simulink model "sl_quadcopter_tres_poster"  (R2014a)
settings: Solver=ode45  StartTime=0.0  StopTime=20  MaxStep=0.1  RelTol=1e-3
InitFcn:
  | % load parameters of the default quadrotor
  | disp('Quadrotor parameters loaded by InitFcn')
  | mdl_quadcopter
undefined symbols (not defined in the file or in its folder): quad
libraries: tres_simulink_blockset x5, roblocks x2
settings Model: Creator=corkep  LastModifiedBy=matteo
settings DataIOCC: SignalLoggingSaveFormat=ModelDataLogs
settings OptimizationCC: ExpressionDepthLimit=2147483647
settings DebuggingCC: UnderspecifiedInitializationDetection=Classic  FcnCallInpInsideContextMsg=EnableAllAsWarning  StateNameClashWarn=warning
settings GRTTargetCC: CombineOutputUpdateFcns=off  GRTInterface=on

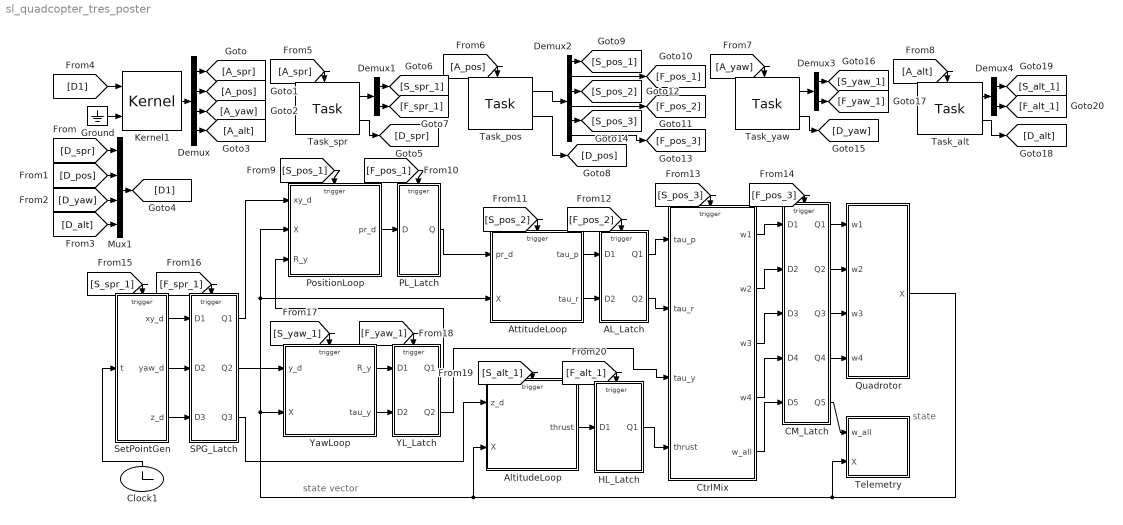
== system sl_quadcopter_tres_poster ==
  note: state
  note: state vector
  AL_Latch : Subsystem  TreatAsAtomicUnit=on
  AltitudeLoop : Subsystem
  AttitudeLoop : Subsystem
  CM_Latch : Subsystem  TreatAsAtomicUnit=on
  Clock1 : Clock
  CtrlMix : Subsystem
  Demux : Demux
  Demux1 : Demux  Outputs=2
  Demux2 : Demux  Outputs=6
  Demux3 : Demux  Outputs=2
  Demux4 : Demux  Outputs=2
  Ground : Ground
  HL_Latch : Subsystem  TreatAsAtomicUnit=on
  Kernel1 : tres_simulink_blockset/Kernel  taskset_descr_name=task_set_descr  scheduling_policy=FIXED_PRIORITY  dead_miss_rule=Continue  time_res=Milli_Seconds  core_num=1  under_engine=RTSIM
  Mux1 : Mux
  PL_Latch : Subsystem  TreatAsAtomicUnit=on
  PositionLoop : Subsystem
  Quadrotor : Subsystem
  SPG_Latch : Subsystem  TreatAsAtomicUnit=on
  SetPointGen : Subsystem
  Task_alt : tres_simulink_blockset/Task  conf_name=alt_instrs
  Task_pos : tres_simulink_blockset/Task  conf_name=att_instrs
  Task_spr : tres_simulink_blockset/Task  conf_name=spr_instrs
  Task_yaw : tres_simulink_blockset/Task  conf_name=yaw_instrs
  Telemetry : Subsystem
  YL_Latch : Subsystem  TreatAsAtomicUnit=on
  YawLoop : Subsystem
  wires:
  SetPointGen/1(xy_d) -> SPG_Latch/1(D1)
  Clock1/1 -> SetPointGen/1(t)
  SetPointGen/2(yaw_d) -> SPG_Latch/2(D2)
  SetPointGen/3(z_d) -> SPG_Latch/3(D3)
  SPG_Latch/1(Q1) -> PositionLoop/1(xy_d)
  SPG_Latch/2(Q2) -> YawLoop/1(y_d)
  SPG_Latch/3(Q3) -> AltitudeLoop/1(z_d)
  YawLoop/1(R_y) -> YL_Latch/1(D1)
  YL_Latch/1(Q1) -> PositionLoop/3(R_y)
  YawLoop/2(tau_y) -> YL_Latch/2(D2)
  YL_Latch/2(Q2) -> CtrlMix/3(tau_y)
  AltitudeLoop/1(thrust) -> HL_Latch/1(D1)
  HL_Latch/1(Q1) -> CtrlMix/4(thrust)
  PositionLoop/1(pr_d) -> PL_Latch/1(D)
  PL_Latch/1(Q) -> AttitudeLoop/1(pr_d)
  AttitudeLoop/1(tau_p) -> AL_Latch/1(D1)
  AttitudeLoop/2(tau_r) -> AL_Latch/2(D2)
  AL_Latch/1(Q1) -> CtrlMix/1(tau_p)
  AL_Latch/2(Q2) -> CtrlMix/2(tau_r)
  CtrlMix/1(w1) -> CM_Latch/1(D1)
  CtrlMix/2(w2) -> CM_Latch/2(D2)
  CtrlMix/3(w3) -> CM_Latch/3(D3)
  CtrlMix/4(w4) -> CM_Latch/4(D4)
  CtrlMix/5(w_all) -> CM_Latch/5(D5)
  CM_Latch/5(Q5) -> Telemetry/1(w_all)
  Ground/1 -> Kernel1/2
  [D_spr] -> Mux1/1
  [D_pos] -> Mux1/2
  [D_yaw] -> Mux1/3
  [D_alt] -> Mux1/4
  Kernel1/1 -> Demux/1
  Demux/1 -> [A_spr]
  Demux/2 -> [A_pos]
  Demux/3 -> [A_yaw]
  Demux/4 -> [A_alt]
  Mux1/1 -> [D1]
  [D1] -> Kernel1/1
  [A_spr] -> Task_spr/Trigger
  Task_spr/1 -> Demux1/1
  Task_spr/2 -> [D_spr]
  Demux1/1 -> [S_spr_1]
  Demux1/2 -> [F_spr_1]
  [A_pos] -> Task_pos/Trigger
  Task_pos/1 -> Demux2/1
  Task_pos/2 -> [D_pos]
  Demux2/1 -> [S_pos_1]
  Demux2/2 -> [F_pos_1]
  Demux2/3 -> [S_pos_2]
  Demux2/4 -> [F_pos_2]
  Demux2/5 -> [S_pos_3]
  Demux2/6 -> [F_pos_3]
  [A_yaw] -> Task_yaw/Trigger
  Task_yaw/1 -> Demux3/1
  Task_yaw/2 -> [D_yaw]
  Demux3/1 -> [S_yaw_1]
  Demux3/2 -> [F_yaw_1]
  [A_alt] -> Task_alt/Trigger
  Task_alt/1 -> Demux4/1
  Task_alt/2 -> [D_alt]
  Demux4/1 -> [S_alt_1]
  Demux4/2 -> [F_alt_1]
  [S_pos_1] -> PositionLoop/Trigger
  [F_pos_1] -> PL_Latch/Trigger
  [F_pos_2] -> AL_Latch/Trigger
  [S_pos_2] -> AttitudeLoop/Trigger
  [S_yaw_1] -> YawLoop/Trigger
  [F_yaw_1] -> YL_Latch/Trigger
  [S_spr_1] -> SetPointGen/Trigger
  [F_spr_1] -> SPG_Latch/Trigger
  [S_pos_3] -> CtrlMix/Trigger
  [F_pos_3] -> CM_Latch/Trigger
  [S_alt_1] -> AltitudeLoop/Trigger
  [F_alt_1] -> HL_Latch/Trigger
  Quadrotor/1(X) -> Telemetry/2(X), YawLoop/2(X), AttitudeLoop/2(X), PositionLoop/2(X), AltitudeLoop/2(X)
  CM_Latch/1(Q1) -> Quadrotor/1(w1)
  CM_Latch/2(Q2) -> Quadrotor/2(w2)
  CM_Latch/3(Q3) -> Quadrotor/3(w3)
  CM_Latch/4(Q4) -> Quadrotor/4(w4)

== system sl_quadcopter_tres_poster/AL_Latch ==
  D1 : Inport
  D2 : Inport  Port=2
  function : TriggerPort  TriggerType=function-call
  Q1 : Outport
  Q2 : Outport  Port=2
  wires:
  D1/1 -> Q1/1
  D2/1 -> Q2/1

== system sl_quadcopter_tres_poster/AltitudeLoop ==
  z_d : Inport
  X : Inport  Port=2
  function : TriggerPort  TriggerType=function-call  PortDimensions=1
  Subsystem : Subsystem
  thrust : Outport
  wires:
  X/1 -> Subsystem/2(In2)
  z_d/1 -> Subsystem/1(In1)
  Subsystem/1(Out1) -> thrust/1

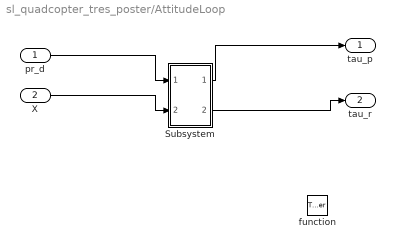
== system sl_quadcopter_tres_poster/AttitudeLoop ==
  pr_d : Inport
  X : Inport  Port=2
  function : TriggerPort  TriggerType=function-call  PortDimensions=1
  Subsystem : Subsystem
  tau_p : Outport
  tau_r : Outport  Port=2
  wires:
  Subsystem/1(Out1) -> tau_p/1
  pr_d/1 -> Subsystem/1(In1)
  Subsystem/2(Out2) -> tau_r/1
  X/1 -> Subsystem/2(In2)

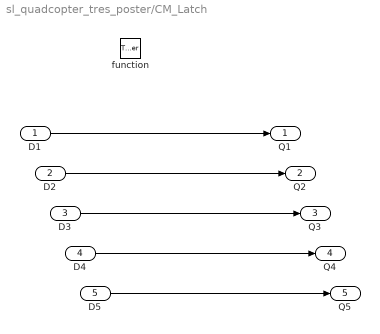
== system sl_quadcopter_tres_poster/CM_Latch ==
  D1 : Inport
  D2 : Inport  Port=2
  D3 : Inport  Port=3
  D4 : Inport  Port=4
  D5 : Inport  Port=5
  function : TriggerPort  TriggerType=function-call
  Q1 : Outport
  Q2 : Outport  Port=2
  Q3 : Outport  Port=3
  Q4 : Outport  Port=4
  Q5 : Outport  Port=5
  wires:
  D1/1 -> Q1/1
  D2/1 -> Q2/1
  D3/1 -> Q3/1
  D4/1 -> Q4/1
  D5/1 -> Q5/1

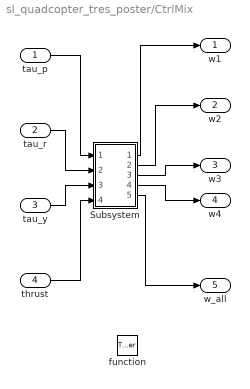
== system sl_quadcopter_tres_poster/CtrlMix ==
  tau_p : Inport
  tau_r : Inport  Port=2
  tau_y : Inport  Port=3
  thrust : Inport  Port=4
  function : TriggerPort  TriggerType=function-call  PortDimensions=1
  Subsystem : Subsystem
  w1 : Outport
  w2 : Outport  Port=2
  w3 : Outport  Port=3
  w4 : Outport  Port=4
  w_all : Outport  Port=5
  wires:
  Subsystem/1(Out1) -> w1/1
  tau_p/1 -> Subsystem/1(In1)
  Subsystem/2(Out2) -> w2/1
  tau_r/1 -> Subsystem/2(In2)
  Subsystem/3(Out3) -> w3/1
  tau_y/1 -> Subsystem/3(In3)
  Subsystem/4(Out4) -> w4/1
  thrust/1 -> Subsystem/4(In4)
  Subsystem/5(Out5) -> w_all/1

== system sl_quadcopter_tres_poster/HL_Latch ==
  D1 : Inport
  function : TriggerPort  TriggerType=function-call
  Q1 : Outport
  wires:
  D1/1 -> Q1/1

== system sl_quadcopter_tres_poster/PL_Latch ==
  D : Inport
  function : TriggerPort  TriggerType=function-call
  Q : Outport
  wires:
  D/1 -> Q/1

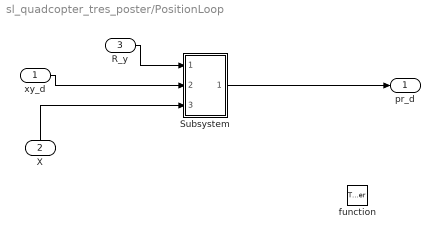
== system sl_quadcopter_tres_poster/PositionLoop ==
  xy_d : Inport
  X : Inport  Port=2
  R_y : Inport  Port=3
  function : TriggerPort  TriggerType=function-call  PortDimensions=1
  Subsystem : Subsystem
  pr_d : Outport
  wires:
  xy_d/1 -> Subsystem/2(In2)
  Subsystem/1(Out1) -> pr_d/1
  R_y/1 -> Subsystem/1(R_y)
  X/1 -> Subsystem/3(In3)

== system sl_quadcopter_tres_poster/Quadrotor ==
  w1 : Inport
  w2 : Inport  Port=2
  w3 : Inport  Port=3
  w4 : Inport  Port=4
  Quadrotor : roblocks/Dynamics/Quadrotor  quad=quad
  X : Outport
  wires:
  w1/1 -> Quadrotor/1
  w2/1 -> Quadrotor/2
  w3/1 -> Quadrotor/3
  w4/1 -> Quadrotor/4
  Quadrotor/1 -> X/1

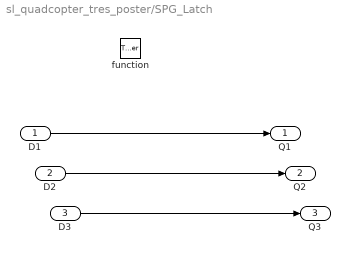
== system sl_quadcopter_tres_poster/SPG_Latch ==
  D1 : Inport
  D2 : Inport  Port=2
  D3 : Inport  Port=3
  function : TriggerPort  TriggerType=function-call
  Q1 : Outport
  Q2 : Outport  Port=2
  Q3 : Outport  Port=3
  wires:
  D1/1 -> Q1/1
  D2/1 -> Q2/1
  D3/1 -> Q3/1

== system sl_quadcopter_tres_poster/SetPointGen ==
  t : Inport
  function : TriggerPort  TriggerType=function-call  PortDimensions=1
  Subsystem : Subsystem
  xy_d : Outport
  yaw_d : Outport  Port=2
  z_d : Outport  Port=3
  wires:
  Subsystem/1(Out1) -> xy_d/1
  Subsystem/3(Out3) -> z_d/1
  t/1 -> Subsystem/1(In1)
  Subsystem/2(Out2) -> yaw_d/1

== system sl_quadcopter_tres_poster/Telemetry ==
  w_all : Inport
  X : Inport  Port=2
  Clock : Clock
  Mux : Mux  Inputs=3
  To Workspace : ToWorkspace  VariableName=result_tres  SampleTime=0.05
  wires:
  Mux/1 -> To Workspace/1
  Clock/1 -> Mux/1
  X/1 -> Mux/2
  w_all/1 -> Mux/3

== system sl_quadcopter_tres_poster/YL_Latch ==
  D1 : Inport
  D2 : Inport  Port=2
  function : TriggerPort  TriggerType=function-call
  Q1 : Outport
  Q2 : Outport  Port=2
  wires:
  D1/1 -> Q1/1
  D2/1 -> Q2/1

== system sl_quadcopter_tres_poster/YawLoop ==
  y_d : Inport
  X : Inport  Port=2
  function : TriggerPort  TriggerType=function-call  PortDimensions=1
  Subsystem : Subsystem
  R_y : Outport
  tau_y : Outport  Port=2
  wires:
  X/1 -> Subsystem/2(In2)
  Subsystem/1(Out1) -> R_y/1
  y_d/1 -> Subsystem/1(In1)
  Subsystem/2(Out2) -> tau_y/1

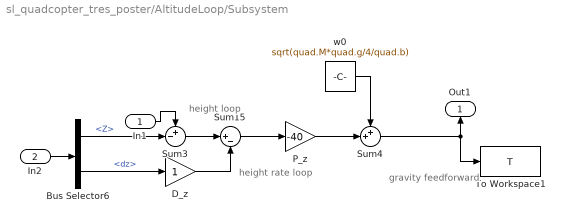
== system sl_quadcopter_tres_poster/AltitudeLoop/Subsystem ==
  note: gravity feedforward
  note: height rate
      | loop
  note: height
      | loop
  In1 : Inport
  In2 : Inport  Port=2
  Bus Selector6 : BusSelector  OutputSignals=Z,dz
  D_z : Gain
  P_z : Gain  Gain=-40
  Sum15 : Sum  Inputs=|+-
  Sum3 : Sum  Inputs=+-|
  Sum4 : Sum  Inputs=++|
  To Workspace1 : ToWorkspace  VariableName=T  SampleTime=-1
  w0 : Constant  Value=sqrt(quad.M*quad.g/4/quad.b)  SampleTime=-1
  Out1 : Outport
  wires:
  w0/1 -> Sum4/1
  Sum15/1 -> P_z/1
  P_z/1 -> Sum4/2
  Bus Selector6/1 -> Sum3/2  "<Z>"
  Sum3/1 -> Sum15/1
  Bus Selector6/2 -> D_z/1  "<dz>"
  D_z/1 -> Sum15/2
  Sum4/1 -> To Workspace1/1, Out1/1
  In1/1 -> Sum3/1
  In2/1 -> Bus Selector6/1

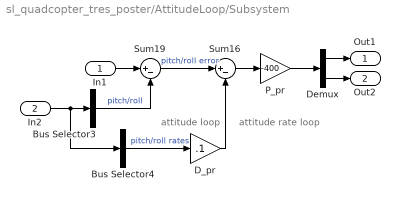
== system sl_quadcopter_tres_poster/AttitudeLoop/Subsystem ==
  note: attitude rate
      | loop
  note: attitude
      | loop
  In1 : Inport
  In2 : Inport  Port=2
  Bus Selector3 : BusSelector  OutputSignals=pitch,roll  OutputAsBus=on
  Bus Selector4 : BusSelector  OutputSignals=dpitch,droll  OutputAsBus=on
  D_pr : Gain  Gain=.1
  Demux : Demux  Outputs=2
  P_pr : Gain  Gain=-400
  Sum16 : Sum  Inputs=|+-
  Sum19 : Sum  Inputs=|+-
  Out1 : Outport
  Out2 : Outport  Port=2
  wires:
  Bus Selector3/1 -> Sum19/2  "pitch/roll"
  Bus Selector4/1 -> D_pr/1  "pitch/roll rates"
  Sum19/1 -> Sum16/1  "pitch/roll error"
  Sum16/1 -> P_pr/1
  P_pr/1 -> Demux/1
  D_pr/1 -> Sum16/2
  In2/1 -> Bus Selector3/1, Bus Selector4/1
  Demux/1 -> Out1/1
  In1/1 -> Sum19/1
  Demux/2 -> Out2/1

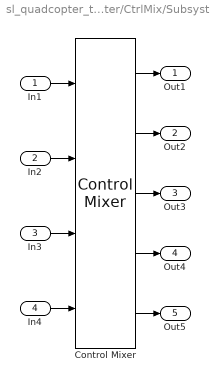
== system sl_quadcopter_tres_poster/CtrlMix/Subsystem ==
  In1 : Inport
  In2 : Inport  Port=2
  In3 : Inport  Port=3
  In4 : Inport  Port=4
  Control Mixer : roblocks/Dynamics/Control Mixer
  Out1 : Outport
  Out2 : Outport  Port=2
  Out3 : Outport  Port=3
  Out4 : Outport  Port=4
  Out5 : Outport  Port=5
  wires:
  Control Mixer/1 -> Out1/1
  In1/1 -> Control Mixer/1
  Control Mixer/2 -> Out2/1
  In2/1 -> Control Mixer/2
  Control Mixer/3 -> Out3/1
  In3/1 -> Control Mixer/3
  Control Mixer/4 -> Out4/1
  In4/1 -> Control Mixer/4
  Control Mixer/5 -> Out5/1

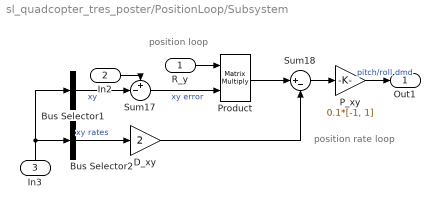
== system sl_quadcopter_tres_poster/PositionLoop/Subsystem ==
  note: position rate
      | loop
  note: position
      | loop
  R_y : Inport
  In2 : Inport  Port=2
  In3 : Inport  Port=3
  Bus Selector1 : BusSelector  OutputSignals=X,Y  OutputAsBus=on
  Bus Selector2 : BusSelector  OutputSignals=dx,dy  OutputAsBus=on
  D_xy : Gain  Gain=2
  P_xy : Gain  Gain=0.1*[-1, 1]
  Product : Product  Multiplication=Matrix(*)  RndMeth=Zero
  Sum17 : Sum  Inputs=+-|
  Sum18 : Sum  Inputs=|+-
  Out1 : Outport
  wires:
  Bus Selector1/1 -> Sum17/2  "xy"
  Bus Selector2/1 -> D_xy/1  "xy rates"
  D_xy/1 -> Sum18/2
  Sum18/1 -> P_xy/1
  Product/1 -> Sum18/1
  Sum17/1 -> Product/2  "xy error"
  In3/1 -> Bus Selector1/1, Bus Selector2/1
  R_y/1 -> Product/1
  In2/1 -> Sum17/1
  P_xy/1 -> Out1/1  "pitch/roll dmd"

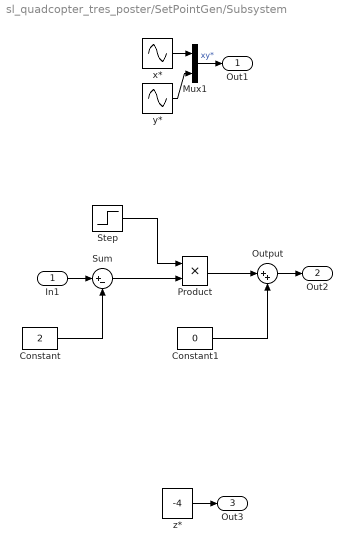
== system sl_quadcopter_tres_poster/SetPointGen/Subsystem ==
  In1 : Inport
  Constant : Constant  DisableCoverage=on  Value=2  OutDataTypeStr=Inherit: Inherit via back propagation
  Constant1 : Constant  DisableCoverage=on  Value=0  OutDataTypeStr=Inherit: Inherit via back propagation
  Mux1 : Mux  Inputs=2
  Output : Sum  Inputs=|++  SaturateOnIntegerOverflow=on  InputSameDT=on  OutDataTypeStr=Inherit: Same as first input
  Product : Product  DisableCoverage=on  SaturateOnIntegerOverflow=on  InputSameDT=on  OutDataTypeStr=Inherit: Same as first input
  Step : Step  DisableCoverage=on  Time=2  After=0.2
  Sum : Sum  DisableCoverage=on  Inputs=|+-  SaturateOnIntegerOverflow=on  InputSameDT=on  OutDataTypeStr=Inherit: Same as first input
  x* : Sin  Frequency=2*pi*.125  Phase=-pi/2
  y* : Sin  Frequency=2*pi*.125
  z* : Constant  Value=-4
  Out1 : Outport
  Out2 : Outport  Port=2
  Out3 : Outport  Port=3
  wires:
  x*/1 -> Mux1/1
  y*/1 -> Mux1/2
  Constant/1 -> Sum/2
  Sum/1 -> Product/2
  Constant1/1 -> Output/2
  Product/1 -> Output/1
  Step/1 -> Product/1
  Mux1/1 -> Out1/1  "xy*"
  Output/1 -> Out2/1
  In1/1 -> Sum/1
  z*/1 -> Out3/1

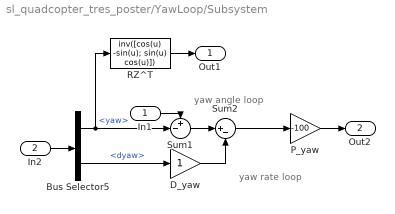
== system sl_quadcopter_tres_poster/YawLoop/Subsystem ==
  note: yaw rate
      | loop
  note: yaw angle
      | loop
  In1 : Inport
  In2 : Inport  Port=2
  Bus Selector5 : BusSelector  OutputSignals=yaw,dyaw
  D_yaw : Gain
  P_yaw : Gain  Gain=-100
  RZ^T : MATLABFcn  MATLABFcn=inv([cos(u) -sin(u); sin(u) cos(u)])  OutputDimensions=[2 2]  Output1D=off
  Sum1 : Sum  Inputs=+-|
  Sum2 : Sum  Inputs=|+-
  Out1 : Outport
  Out2 : Outport  Port=2
  wires:
  Bus Selector5/1 -> RZ^T/1, Sum1/2  "<yaw>"
  Sum2/1 -> P_yaw/1
  Bus Selector5/2 -> D_yaw/1  "<dyaw>"
  D_yaw/1 -> Sum2/2
  Sum1/1 -> Sum2/1
  RZ^T/1 -> Out1/1
  In1/1 -> Sum1/1
  P_yaw/1 -> Out2/1
  In2/1 -> Bus Selector5/1
